simulink model "soccer"
settings: Solver=ode45  StartTime=0.0  StopTime=150  RelTol=1e-3
PostLoadFcn:
  | init_motes
InitFcn:
  | clear functions
undefined symbols (not defined in the file): clock, WLAN, xBall, xPos, yBall, yPos
libraries: truetime x11
settings Model: ExtModeAutoUpdateStatusClock=off  Creator=anton  LastModifiedBy=anton
settings DataIOCC: LimitDataPoints=on  SaveFormat=Array  SaveOutput=off  SaveTime=off  ReturnWorkspaceOutputs=off
settings OptimizationCC: BlockReduction=off  BooleanDataType=off  ExpressionDepthLimit=2147483647  LifeSpan=inf  SimCompilerOptimization=Off
settings DebuggingCC: SaveWithParameterizedLinksMsg=none  UnderspecifiedInitializationDetection=Classic  MergeDetectMultiDrivingBlocksExec=none  SignalResolutionControl=TryResolveAllWithWarning  MultiTaskDSMMsg=warning  MultiTaskCondExecSysMsg=none  FcnCallInpInsideContextMsg=Enable All  StateNameClashWarn=warning  SFUnexpectedBacktrackingDiag=warning  SFNoUnconditionalDefaultTransitionDiag=warning
settings HardwareCC: ProdBitPerPointer=32  ProdLargestAtomicFloat=None  ProdIntDivRoundTo=Undefined  ProdEndianess=Unspecified  ProdWordSize=32  ProdHWDeviceType=32-bit Generic  TargetUnknown=on
settings ModelReferenceCC: PropagateSignalLabelsOutOfModel=off
settings SFSimCC: SimUseLocalCustomCode=off
settings RTWCC: RTWUseLocalCustomCode=off  RTWCompilerOptimization=Off
settings GRTTargetCC: TargetFcnLib=ansi_tfl_tmw.mat  CodeReplacementLibrary=C89/C90 (ANSI)  GeneratePreprocessorConditionals=Disable all  CombineOutputUpdateFcns=off  CPPClassGenCompliant=off  GRTInterface=on

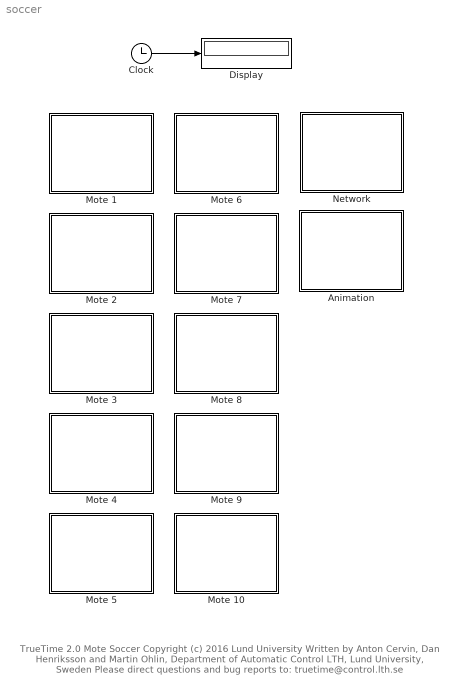
== system soccer ==
  note: TrueTime 2.0  Mote Soccer
      | Copyright (c) 2016 Lund University
      | Written by Anton Cervin, Dan Henriksson and Martin Ohlin,
      | Department of Automatic Control LTH, Lund University, Sweden
      | Please direct questions and bug reports to: truetime@control.lth.se
  Animation : Subsystem  mask{N=10}
      mask prompts: N "Number of nodes"
      mask init:
      | soccer_callback(gcb,N)
  Clock : Clock
  Display : Display
  Mote 1 : Subsystem  mask(fgdfgMOTE){nodeID=1}
      mask prompts: nodeID "Node number"
      mask init:
      | mote_callback(gcb,nodeID)
  Mote 10 : Subsystem  mask(fgdfgMOTE){nodeID=10}
      mask prompts: nodeID "Node number"
      mask init:
      | mote_callback(gcb,nodeID)
  Mote 2 : Subsystem  mask(fgdfgMOTE){nodeID=2}
      mask prompts: nodeID "Node number"
      mask init:
      | mote_callback(gcb,nodeID)
  Mote 3 : Subsystem  mask(fgdfgMOTE){nodeID=3}
      mask prompts: nodeID "Node number"
      mask init:
      | mote_callback(gcb,nodeID)
  Mote 4 : Subsystem  mask(fgdfgMOTE){nodeID=4}
      mask prompts: nodeID "Node number"
      mask init:
      | mote_callback(gcb,nodeID)
  Mote 5 : Subsystem  mask(fgdfgMOTE){nodeID=5}
      mask prompts: nodeID "Node number"
      mask init:
      | mote_callback(gcb,nodeID)
  Mote 6 : Subsystem  mask(fgdfgMOTE){nodeID=6}
      mask prompts: nodeID "Node number"
      mask init:
      | mote_callback(gcb,nodeID)
  Mote 7 : Subsystem  mask(fgdfgMOTE){nodeID=7}
      mask prompts: nodeID "Node number"
      mask init:
      | mote_callback(gcb,nodeID)
  Mote 8 : Subsystem  mask(fgdfgMOTE){nodeID=8}
      mask prompts: nodeID "Node number"
      mask init:
      | mote_callback(gcb,nodeID)
  Mote 9 : Subsystem  mask(fgdfgMOTE){nodeID=9}
      mask prompts: nodeID "Node number"
      mask init:
      | mote_callback(gcb,nodeID)
  Network : Subsystem  mask{N=10}
      mask prompts: N "Number of nodes"
      mask init:
      | soccer_callback(gcb,N)
  wires:
  Clock/1 -> Display/1

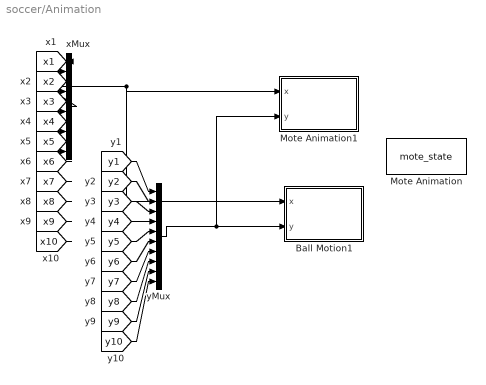
== system soccer/Animation ==
  Ball Motion1 : Subsystem  mask{numMotes=10}
      mask prompts: numMotes "Number of Motes"
  Mote Animation : S-Function  FunctionName=mote_state  EnableBusSupport=off
      settings: DeleteFcn=if ~isempty(findobj('type','figure','name','dblpend1 Animation'));close('dblpend1 Animation'); end;
  Mote Animation1 : Subsystem  mask{numMotes=10, xmax=20, ymax=30, ts=0.1, x0=xPos, y0=yPos}
      mask prompts: numMotes "Number of Motes"; ts "Update period"
  xMux : Mux  Inputs=10
  yMux : Mux  Inputs=10
  wires:
  xMux/1 -> Ball Motion1/1(x), Mote Animation1/1(x)
  yMux/1 -> Mote Animation1/2(y), Ball Motion1/2(y)
  [x1] -> xMux/1
  [y1] -> yMux/1
  [x2] -> xMux/2
  [y2] -> yMux/2
  [x3] -> xMux/3
  [y3] -> yMux/3
  [x4] -> xMux/4
  [y4] -> yMux/4
  [x5] -> xMux/5
  [y5] -> yMux/5
  [x6] -> xMux/6
  [y6] -> yMux/6
  [x7] -> xMux/7
  [y7] -> yMux/7
  [x8] -> xMux/8
  [y8] -> yMux/8
  [x9] -> xMux/9
  [y9] -> yMux/9
  [x10] -> xMux/10
  [y10] -> yMux/10

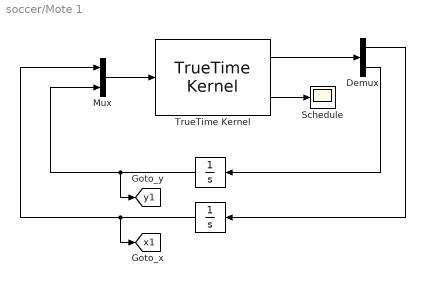
== system soccer/Mote 1 ==
  " " : Integrator  InitialCondition=yPos(nodeID)
  " " : Integrator  InitialCondition=xPos(nodeID)
  Demux : Demux  Outputs=2
  Mux : Mux  Inputs=2
  Schedule : Scope
      settings: TickLabels=on  TimeRange=3.5  YMin=1.8  YMax=3.7
  TrueTime Kernel : truetime/TrueTime Kernel  sfun=node_red_goalie_init  args=nodeID  ninputsoutputs=[2 2]  ntriggers=0  trigtype=falling  nwnodenbr=nodeID  clockoffsetdrift=[0 0]  schedoutput=on  battery=off  poweroutput=off  label=1: 1
  tag scope: x1=global, y1=global
  wires:
  TrueTime Kernel/1 -> Demux/1
  Demux/2 -> " "/1
  Demux/1 -> " "/1
  " "/1 -> Mux/2, [y1]
  " "/1 -> Mux/1, [x1]
  Mux/1 -> TrueTime Kernel/1
  TrueTime Kernel/2 -> Schedule/1

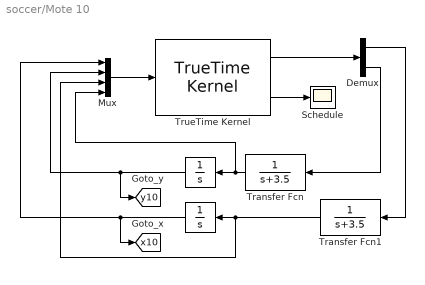
== system soccer/Mote 10 ==
  " " : Integrator  InitialCondition=yPos(nodeID)
  " " : Integrator  InitialCondition=xPos(nodeID)
  Demux : Demux  Outputs=2
  Mux : Mux
  Schedule : Scope
      settings: TickLabels=on  TimeRange=3.5  YMin=1.8  YMax=3.7  SaveName=ScopeData2
  Transfer Fcn : TransferFcn  Denominator=[1 3.5]
  Transfer Fcn1 : TransferFcn  Denominator=[1 3.5]
  TrueTime Kernel : truetime/TrueTime Kernel  sfun=node_blue_init  args=nodeID  ninputsoutputs=[4 2]  ntriggers=0  trigtype=falling  nwnodenbr=nodeID  clockoffsetdrift=[0 0]  schedoutput=on  battery=off  poweroutput=off  label=1: 10
  tag scope: x10=global, y10=global
  wires:
  TrueTime Kernel/1 -> Demux/1
  Demux/2 -> Transfer Fcn/1
  Demux/1 -> Transfer Fcn1/1
  " "/1 -> Mux/2, [y10]
  " "/1 -> Mux/1, [x10]
  Transfer Fcn/1 -> " "/1, Mux/4
  Transfer Fcn1/1 -> " "/1, Mux/3
  Mux/1 -> TrueTime Kernel/1
  TrueTime Kernel/2 -> Schedule/1

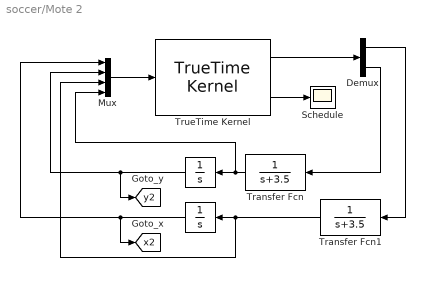
== system soccer/Mote 2 ==
  " " : Integrator  InitialCondition=yPos(nodeID)
  " " : Integrator  InitialCondition=xPos(nodeID)
  Demux : Demux  Outputs=2
  Mux : Mux
  Schedule : Scope
      settings: TickLabels=on  TimeRange=3.5  YMin=1.8  YMax=3.7
  Transfer Fcn : TransferFcn  Denominator=[1 3.5]
  Transfer Fcn1 : TransferFcn  Denominator=[1 3.5]
  TrueTime Kernel : truetime/TrueTime Kernel  sfun=node_red_init  args=nodeID  ninputsoutputs=[4 2]  ntriggers=0  trigtype=falling  nwnodenbr=nodeID  clockoffsetdrift=[0 0]  schedoutput=on  battery=off  poweroutput=off  label=1: 2
  tag scope: x2=global, y2=global
  wires:
  TrueTime Kernel/1 -> Demux/1
  Demux/2 -> Transfer Fcn/1
  Demux/1 -> Transfer Fcn1/1
  " "/1 -> Mux/2, [y2]
  " "/1 -> Mux/1, [x2]
  Transfer Fcn/1 -> " "/1, Mux/4
  Transfer Fcn1/1 -> " "/1, Mux/3
  Mux/1 -> TrueTime Kernel/1
  TrueTime Kernel/2 -> Schedule/1

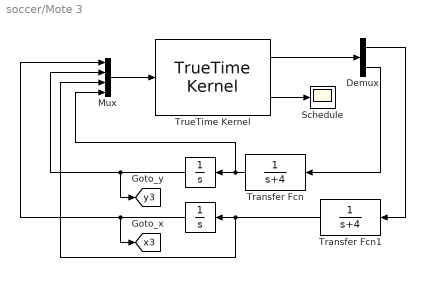
== system soccer/Mote 3 ==
  " " : Integrator  InitialCondition=yPos(nodeID)
  " " : Integrator  InitialCondition=xPos(nodeID)
  Demux : Demux  Outputs=2
  Mux : Mux
  Schedule : Scope
      settings: TickLabels=on  TimeRange=3.5  YMin=1.8  YMax=3.7
  Transfer Fcn : TransferFcn  Denominator=[1 4]
  Transfer Fcn1 : TransferFcn  Denominator=[1 4]
  TrueTime Kernel : truetime/TrueTime Kernel  sfun=node_red_init  args=nodeID  ninputsoutputs=[4 2]  ntriggers=0  trigtype=falling  nwnodenbr=nodeID  clockoffsetdrift=[0 0]  schedoutput=on  battery=off  poweroutput=off  label=1: 3
  tag scope: x3=global, y3=global
  wires:
  TrueTime Kernel/2 -> Schedule/1
  Mux/1 -> TrueTime Kernel/1
  Transfer Fcn1/1 -> Mux/3, " "/1
  Transfer Fcn/1 -> Mux/4, " "/1
  " "/1 -> [x3], Mux/1
  " "/1 -> [y3], Mux/2
  Demux/1 -> Transfer Fcn1/1
  Demux/2 -> Transfer Fcn/1
  TrueTime Kernel/1 -> Demux/1

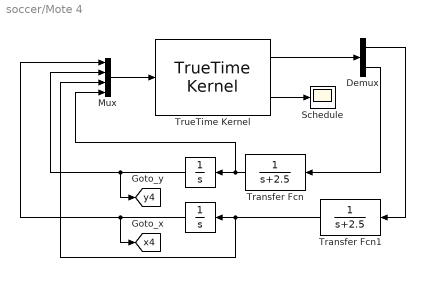
== system soccer/Mote 4 ==
  " " : Integrator  InitialCondition=yPos(nodeID)
  " " : Integrator  InitialCondition=xPos(nodeID)
  Demux : Demux  Outputs=2
  Mux : Mux
  Schedule : Scope
      settings: TickLabels=on  TimeRange=3.5  YMin=1.8  YMax=3.7
  Transfer Fcn : TransferFcn  Denominator=[1 2.5]
  Transfer Fcn1 : TransferFcn  Denominator=[1 2.5]
  TrueTime Kernel : truetime/TrueTime Kernel  sfun=node_red_init  args=nodeID  ninputsoutputs=[4 2]  ntriggers=0  trigtype=falling  nwnodenbr=nodeID  clockoffsetdrift=[0 0]  schedoutput=on  battery=off  poweroutput=off  label=1: 4
  tag scope: x4=global, y4=global
  wires:
  TrueTime Kernel/1 -> Demux/1
  Demux/2 -> Transfer Fcn/1
  Demux/1 -> Transfer Fcn1/1
  " "/1 -> Mux/2, [y4]
  " "/1 -> Mux/1, [x4]
  Transfer Fcn/1 -> " "/1, Mux/4
  Transfer Fcn1/1 -> " "/1, Mux/3
  Mux/1 -> TrueTime Kernel/1
  TrueTime Kernel/2 -> Schedule/1

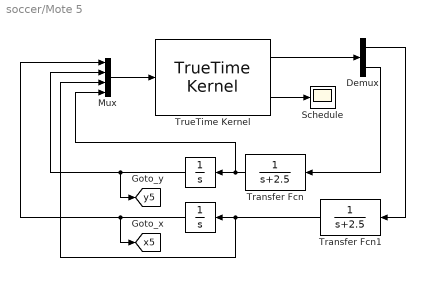
== system soccer/Mote 5 ==
  " " : Integrator  InitialCondition=yPos(nodeID)
  " " : Integrator  InitialCondition=xPos(nodeID)
  Demux : Demux  Outputs=2
  Mux : Mux
  Schedule : Scope
      settings: TickLabels=on  TimeRange=3.5  YMin=1.8  YMax=3.7
  Transfer Fcn : TransferFcn  Denominator=[1 2.5]
  Transfer Fcn1 : TransferFcn  Denominator=[1 2.5]
  TrueTime Kernel : truetime/TrueTime Kernel  sfun=node_red_init  args=nodeID  ninputsoutputs=[4 2]  ntriggers=0  trigtype=falling  nwnodenbr=nodeID  clockoffsetdrift=[0 0]  schedoutput=on  battery=off  poweroutput=off  label=1: 5
  tag scope: x5=global, y5=global
  wires:
  TrueTime Kernel/2 -> Schedule/1
  Mux/1 -> TrueTime Kernel/1
  Transfer Fcn1/1 -> Mux/3, " "/1
  Transfer Fcn/1 -> Mux/4, " "/1
  " "/1 -> [x5], Mux/1
  " "/1 -> [y5], Mux/2
  Demux/1 -> Transfer Fcn1/1
  Demux/2 -> Transfer Fcn/1
  TrueTime Kernel/1 -> Demux/1

== system soccer/Mote 6 ==
  " " : Integrator  InitialCondition=yPos(nodeID)
  " " : Integrator  InitialCondition=xPos(nodeID)
  Demux : Demux  Outputs=2
  Mux : Mux  Inputs=2
  Schedule : Scope
      settings: TickLabels=on  TimeRange=3.5  YMin=1.8  YMax=3.7
  TrueTime Kernel : truetime/TrueTime Kernel  sfun=node_blue_goalie_init  args=nodeID  ninputsoutputs=[2 2]  ntriggers=0  trigtype=falling  nwnodenbr=nodeID  clockoffsetdrift=[0 0]  schedoutput=on  battery=off  poweroutput=off  label=1: 6
  tag scope: x6=global, y6=global
  wires:
  TrueTime Kernel/1 -> Demux/1
  Demux/2 -> " "/1
  Demux/1 -> " "/1
  " "/1 -> Mux/2, [y6]
  " "/1 -> Mux/1, [x6]
  Mux/1 -> TrueTime Kernel/1
  TrueTime Kernel/2 -> Schedule/1

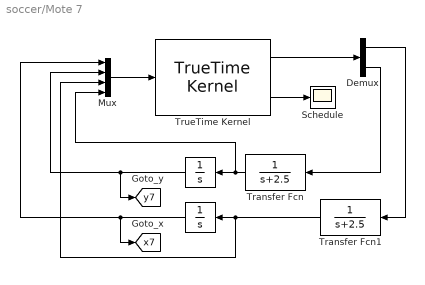
== system soccer/Mote 7 ==
  " " : Integrator  InitialCondition=yPos(nodeID)
  " " : Integrator  InitialCondition=xPos(nodeID)
  Demux : Demux  Outputs=2
  Mux : Mux
  Schedule : Scope
      settings: TickLabels=on  TimeRange=3.5  YMin=1.8  YMax=3.7  SaveName=ScopeData2
  Transfer Fcn : TransferFcn  Denominator=[1 2.5]
  Transfer Fcn1 : TransferFcn  Denominator=[1 2.5]
  TrueTime Kernel : truetime/TrueTime Kernel  sfun=node_blue_init  args=nodeID  ninputsoutputs=[4 2]  ntriggers=0  trigtype=falling  nwnodenbr=nodeID  clockoffsetdrift=[0 0]  schedoutput=on  battery=off  poweroutput=off  label=1: 7
  tag scope: x7=global, y7=global
  wires:
  TrueTime Kernel/1 -> Demux/1
  Demux/2 -> Transfer Fcn/1
  Demux/1 -> Transfer Fcn1/1
  " "/1 -> Mux/2, [y7]
  " "/1 -> Mux/1, [x7]
  Transfer Fcn/1 -> " "/1, Mux/4
  Transfer Fcn1/1 -> " "/1, Mux/3
  Mux/1 -> TrueTime Kernel/1
  TrueTime Kernel/2 -> Schedule/1

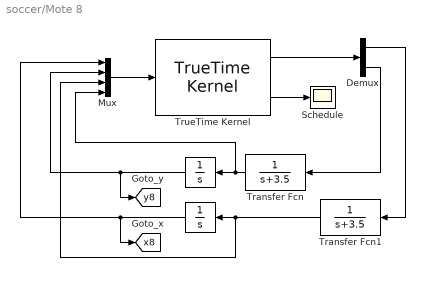
== system soccer/Mote 8 ==
  " " : Integrator  InitialCondition=yPos(nodeID)
  " " : Integrator  InitialCondition=xPos(nodeID)
  Demux : Demux  Outputs=2
  Mux : Mux
  Schedule : Scope
      settings: TickLabels=on  TimeRange=3.5  YMin=1.8  YMax=3.7  SaveName=ScopeData2
  Transfer Fcn : TransferFcn  Denominator=[1 3.5]
  Transfer Fcn1 : TransferFcn  Denominator=[1 3.5]
  TrueTime Kernel : truetime/TrueTime Kernel  sfun=node_blue_init  args=nodeID  ninputsoutputs=[4 2]  ntriggers=0  trigtype=falling  nwnodenbr=nodeID  clockoffsetdrift=[0 0]  schedoutput=on  battery=off  poweroutput=off  label=1: 8
  tag scope: x8=global, y8=global
  wires:
  TrueTime Kernel/1 -> Demux/1
  Demux/2 -> Transfer Fcn/1
  Demux/1 -> Transfer Fcn1/1
  " "/1 -> Mux/2, [y8]
  " "/1 -> Mux/1, [x8]
  Transfer Fcn/1 -> " "/1, Mux/4
  Transfer Fcn1/1 -> " "/1, Mux/3
  Mux/1 -> TrueTime Kernel/1
  TrueTime Kernel/2 -> Schedule/1

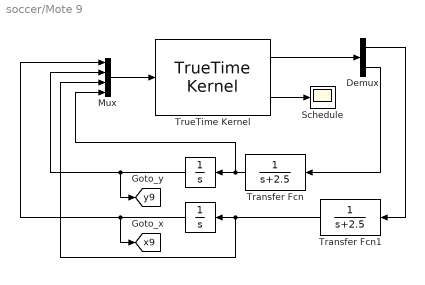
== system soccer/Mote 9 ==
  " " : Integrator  InitialCondition=yPos(nodeID)
  " " : Integrator  InitialCondition=xPos(nodeID)
  Demux : Demux  Outputs=2
  Mux : Mux
  Schedule : Scope
      settings: TickLabels=on  TimeRange=3.5  YMin=1.8  YMax=3.7  SaveName=ScopeData2
  Transfer Fcn : TransferFcn  Denominator=[1 2.5]
  Transfer Fcn1 : TransferFcn  Denominator=[1 2.5]
  TrueTime Kernel : truetime/TrueTime Kernel  sfun=node_blue_init  args=nodeID  ninputsoutputs=[4 2]  ntriggers=0  trigtype=falling  nwnodenbr=nodeID  clockoffsetdrift=[0 0]  schedoutput=on  battery=off  poweroutput=off  label=1: 9
  tag scope: x9=global, y9=global
  wires:
  TrueTime Kernel/1 -> Demux/1
  Demux/2 -> Transfer Fcn/1
  Demux/1 -> Transfer Fcn1/1
  " "/1 -> Mux/2, [y9]
  " "/1 -> Mux/1, [x9]
  Transfer Fcn/1 -> " "/1, Mux/4
  Transfer Fcn1/1 -> " "/1, Mux/3
  Mux/1 -> TrueTime Kernel/1
  TrueTime Kernel/2 -> Schedule/1

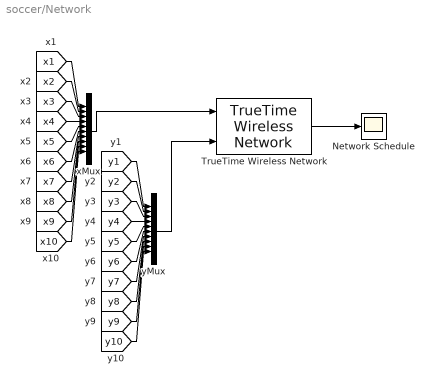
== system soccer/Network ==
  Network Schedule : Scope
      settings: TimeRange=40  YMin=1  YMax=10.5  SaveName=nschedule
  TrueTime Wireless Network : truetime/TrueTime Wireless  Network  nwtype=802.11b (WLAN)  nwnbr=1  nnodes=N  rate=800000  minsize=272  transpower=20  threshold=-48  use_pathloss_function=default  pathloss=3.5  acktimeout=0.00004  retrylimit=5  error_threshold=0.03  lossprob=0  seed=floor(sum(100*clock))  scheduleoutput=on  poweroutput=off
  xMux : Mux  Inputs=10
  yMux : Mux  Inputs=10
  wires:
  xMux/1 -> TrueTime Wireless Network/1
  yMux/1 -> TrueTime Wireless Network/2
  TrueTime Wireless Network/1 -> Network Schedule/1
  [x1] -> xMux/1
  [y1] -> yMux/1
  [x2] -> xMux/2
  [y2] -> yMux/2
  [x3] -> xMux/3
  [y3] -> yMux/3
  [x4] -> xMux/4
  [y4] -> yMux/4
  [x5] -> xMux/5
  [y5] -> yMux/5
  [x6] -> xMux/6
  [y6] -> yMux/6
  [x7] -> xMux/7
  [y7] -> yMux/7
  [x8] -> xMux/8
  [y8] -> yMux/8
  [x9] -> xMux/9
  [y9] -> yMux/9
  [x10] -> xMux/10
  [y10] -> yMux/10

== system soccer/Animation/Ball Motion1 ==
  x : Inport
  y : Inport  Port=2
  Mote Animation : S-Function  FunctionName=ballmotion  Parameters=[numMotes,xBall,yBall]  EnableBusSupport=off
      settings: DeleteFcn=if ~isempty(findobj('type','figure','name','dblpend1 Animation'));close('dblpend1 Animation'); end;
  Mux : Mux  Inputs=2
  wires:
  x/1 -> Mux/1
  y/1 -> Mux/2
  Mux/1 -> Mote Animation/1

== system soccer/Animation/Mote Animation1 ==
  x : Inport
  y : Inport  Port=2
  Mote Animation : S-Function  FunctionName=moteanimation  Parameters=[numMotes ts xmax ymax] x0 y0  EnableBusSupport=off
      settings: DeleteFcn=if ~isempty(findobj('type','figure','name','dblpend1 Animation'));close('dblpend1 Animation'); end;
  Mux : Mux  Inputs=2
  wires:
  Mux/1 -> Mote Animation/1
  y/1 -> Mux/2
  x/1 -> Mux/1
